simulink model "filter_1st_order_iir_cosim"  (Simulink 6.4)
settings: Solver=FixedStepDiscrete  SolverMode=SingleTasking  StartTime=0.0  StopTime=12e-2  RelTol=1e-3
libraries: modelsimlib x1
settings Model: LastModifiedBy=Administrador

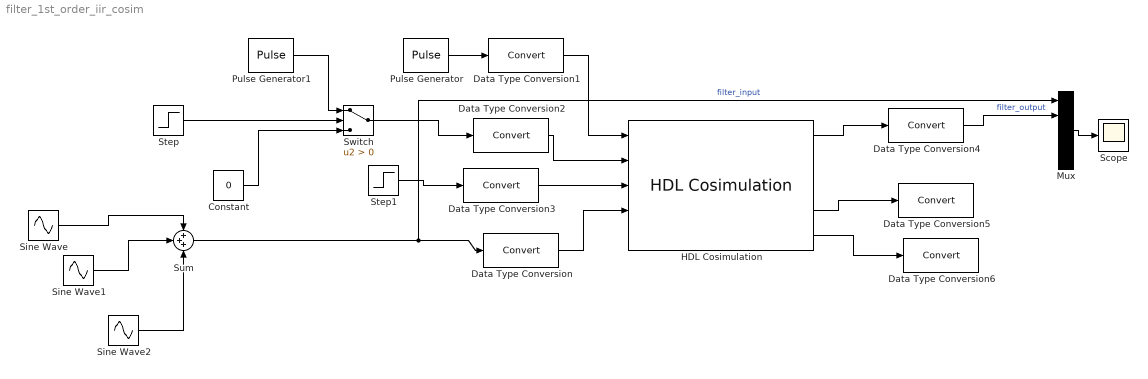
== system filter_1st_order_iir_cosim ==
  Constant : Constant  Value=0  OutDataType=sfix(16)  ConRadixGroup=Use specified scaling  OutScaling=2^0  SampleTime=-1  FramePeriod=inf
  Data Type Conversion : DataTypeConversion  OutDataTypeMode=Specify via dialog  OutScaling=2^(-11)  RndMeth=Nearest  SampleTime=1e-5  SaturateOnIntegerOverflow=on
  Data Type Conversion1 : DataTypeConversion  OutDataTypeMode=boolean
  Data Type Conversion2 : DataTypeConversion  OutDataTypeMode=boolean
  Data Type Conversion3 : DataTypeConversion  OutDataTypeMode=boolean
  Data Type Conversion4 : DataTypeConversion
  Data Type Conversion5 : DataTypeConversion
  Data Type Conversion6 : DataTypeConversion
  HDL Cosimulation : modelsimlib/HDL Cosimulation  DialogController=modelsimddg.CoSim  DialogControllerArgs=DataTag0  PortPaths=/filter_1st_order_iir_cosim_tb/iir_i/clk;/filter_1st_order_iir_cosim_tb/iir_i/run_en;/filter_1st_order_iir_cosim_tb/iir_i/rst;/filter_1st_order_iir_cosim_tb/iir_i/i;/filter_1st_order_iir_cosim_tb/iir_i/o;/filter_1st_order_iir_cosim_tb/iir_i/run_passthru;/filter_1st_order_iir_cosim_tb/iir_i/delayer_in;/filter_1st_order_iir_cosim_tb/iir_i/delayer_out;/filter_1st_order_iir_cosim_tb/iir_i/z1_adder_out_s;/filter_1st_order_iir_cosim_tb/iir_i/b0_mult_out_s  PortModes=[1 1 1 1 2 2 1 2 2 2 ]  PortTimes=[1,1,1,1,1e-5,1,1,1,1e-5,1e-5]  PortSigns=[-1 -1 -1 -1 1 -1 -1 -1 1 1 ]  PortFracLengths=[0,0,0,0,11,0,0,0,11,11]  CommLocal=on  CommSharedMemory=off  CommPortNumber=4449  CommShowInfo=on  ClockModes=[]  ClockTimes=[]  TclPreSimCommand="echo \"Running Simulink Cosimulation block.\""  TclPostSimCommand="echo \"done\""  TimingMode=s  TimingScaleFactor=1  idxCellArray={'UNUSED_VAR'}
  Mux : Mux  Inputs=5
  Pulse Generator : DiscretePulseGenerator  PulseType=Time based  Period=1/(1e6)  PulseWidth=50
  Pulse Generator1 : DiscretePulseGenerator  PulseType=Time based  Period=0.1e-3  PulseWidth=0.5
  Scope : Scope
      settings: YMin=-3  YMax=10  MaxDataPoints=500000
  Sine Wave : Sin  Frequency=2*pi*10  SampleTime=0
  Sine Wave1 : Sin  Frequency=2*pi*50  SampleTime=0
  Sine Wave2 : Sin  Frequency=200*2*pi  SampleTime=0
  Step : Step  Time=4*(1/1e6)
  Step1 : Step  Time=6*(1/1e6)  Before=1  After=0
  Sum : Sum  Inputs=+++
  Switch : Switch  Criteria=u2 > Threshold  RndMeth=Nearest  ZeroCross=off  SampleTime=1e-7
  wires:
  Pulse Generator/1 -> Data Type Conversion1/1
  Data Type Conversion1/1 -> HDL Cosimulation/1
  Switch/1 -> Data Type Conversion2/1
  Data Type Conversion2/1 -> HDL Cosimulation/2
  Step1/1 -> Data Type Conversion3/1
  Constant/1 -> Switch/3
  Step/1 -> Switch/2
  Pulse Generator1/1 -> Switch/1
  Data Type Conversion4/1 -> Mux/2  "filter_output"
  Sum/1 -> Data Type Conversion/1, Mux/1  "filter_input"
  Data Type Conversion3/1 -> HDL Cosimulation/3
  Data Type Conversion/1 -> HDL Cosimulation/4
  HDL Cosimulation/1 -> Data Type Conversion4/1
  Sine Wave/1 -> Sum/1
  HDL Cosimulation/4 -> Data Type Conversion5/1
  HDL Cosimulation/5 -> Data Type Conversion6/1
  Mux/1 -> Scope/1
  Sine Wave1/1 -> Sum/2
  Sine Wave2/1 -> Sum/3
